simulink model "labFinal_5"  (R2018b)
settings: Solver=FixedStepDiscrete  StartTime=0.0  StopTime=10.0  FixedStep=1  RelTol=1e-3
libraries: hdlsllib x2
settings Model: Creator=mllax8  LastModifiedBy=mllax8

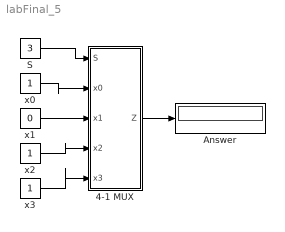
== system labFinal_5 ==
  4-1 MUX : Subsystem
  Answer : Display
  S : Constant  Value=3  OutDataTypeStr=uint8  SampleTime=1
  x0 : Constant  OutDataTypeStr=uint8  SampleTime=1
  x1 : Constant  Value=0  OutDataTypeStr=uint8  SampleTime=1
  x2 : Constant  OutDataTypeStr=uint8  SampleTime=1
  x3 : Constant  OutDataTypeStr=uint8  SampleTime=1
  wires:
  4-1 MUX/1(Z) -> Answer/1
  S/1 -> 4-1 MUX/1(S)
  x0/1 -> 4-1 MUX/2(x0)
  x1/1 -> 4-1 MUX/3(x1)
  x2/1 -> 4-1 MUX/4(x2)
  x3/1 -> 4-1 MUX/5(x3)

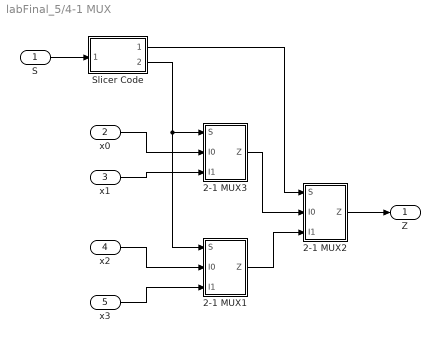
== system labFinal_5/4-1 MUX ==
  S : Inport  OutDataTypeStr=uint8
  x0 : Inport  Port=2  OutDataTypeStr=uint8
  x1 : Inport  Port=3  OutDataTypeStr=uint8
  x2 : Inport  Port=4  OutDataTypeStr=uint8
  x3 : Inport  Port=5  OutDataTypeStr=uint8
  2-1 MUX1 : Subsystem
  2-1 MUX2 : Subsystem
  2-1 MUX3 : Subsystem
  Slicer Code : Subsystem
  Z : Outport
  wires:
  Slicer Code/2("S 2^0 ") -> 2-1 MUX3/1(S), 2-1 MUX1/1(S)
  x0/1 -> 2-1 MUX3/2(I0)
  x1/1 -> 2-1 MUX3/3(I1)
  x2/1 -> 2-1 MUX1/2(I0)
  x3/1 -> 2-1 MUX1/3(I1)
  2-1 MUX3/1(Z) -> 2-1 MUX2/2(I0)
  2-1 MUX1/1(Z) -> 2-1 MUX2/3(I1)
  2-1 MUX2/1(Z) -> Z/1
  S/1 -> Slicer Code/1(uint8)
  Slicer Code/1(S 2^1) -> 2-1 MUX2/1(S)

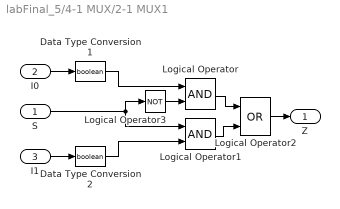
== system labFinal_5/4-1 MUX/2-1 MUX1 ==
  S : Inport
  I0 : Inport  Port=2
  I1 : Inport  Port=3
  Data Type Conversion1 : DataTypeConversion  OutDataTypeStr=boolean
  Data Type Conversion2 : DataTypeConversion  OutDataTypeStr=boolean
  Logical Operator : Logic  AllPortsSameDT=off  OutDataTypeStr=boolean
  Logical Operator1 : Logic  AllPortsSameDT=off  OutDataTypeStr=boolean
  Logical Operator2 : Logic  Operator=OR  AllPortsSameDT=off  OutDataTypeStr=boolean
  Logical Operator3 : Logic  Operator=NOT  AllPortsSameDT=off  OutDataTypeStr=boolean
  Z : Outport
  wires:
  Logical Operator2/1 -> Z/1
  I1/1 -> Data Type Conversion2/1
  Logical Operator1/1 -> Logical Operator2/2
  S/1 -> Logical Operator3/1, Logical Operator1/1
  I0/1 -> Data Type Conversion1/1
  Logical Operator/1 -> Logical Operator2/1
  Data Type Conversion1/1 -> Logical Operator/1
  Data Type Conversion2/1 -> Logical Operator1/2
  Logical Operator3/1 -> Logical Operator/2

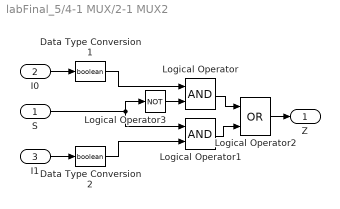
== system labFinal_5/4-1 MUX/2-1 MUX2 ==
  S : Inport
  I0 : Inport  Port=2
  I1 : Inport  Port=3
  Data Type Conversion1 : DataTypeConversion  OutDataTypeStr=boolean
  Data Type Conversion2 : DataTypeConversion  OutDataTypeStr=boolean
  Logical Operator : Logic  AllPortsSameDT=off  OutDataTypeStr=boolean
  Logical Operator1 : Logic  AllPortsSameDT=off  OutDataTypeStr=boolean
  Logical Operator2 : Logic  Operator=OR  AllPortsSameDT=off  OutDataTypeStr=boolean
  Logical Operator3 : Logic  Operator=NOT  AllPortsSameDT=off  OutDataTypeStr=boolean
  Z : Outport
  wires:
  Logical Operator2/1 -> Z/1
  I1/1 -> Data Type Conversion2/1
  Logical Operator1/1 -> Logical Operator2/2
  S/1 -> Logical Operator3/1, Logical Operator1/1
  I0/1 -> Data Type Conversion1/1
  Logical Operator/1 -> Logical Operator2/1
  Data Type Conversion1/1 -> Logical Operator/1
  Data Type Conversion2/1 -> Logical Operator1/2
  Logical Operator3/1 -> Logical Operator/2

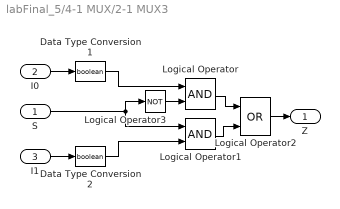
== system labFinal_5/4-1 MUX/2-1 MUX3 ==
  S : Inport
  I0 : Inport  Port=2
  I1 : Inport  Port=3
  Data Type Conversion1 : DataTypeConversion  OutDataTypeStr=boolean
  Data Type Conversion2 : DataTypeConversion  OutDataTypeStr=boolean
  Logical Operator : Logic  AllPortsSameDT=off  OutDataTypeStr=boolean
  Logical Operator1 : Logic  AllPortsSameDT=off  OutDataTypeStr=boolean
  Logical Operator2 : Logic  Operator=OR  AllPortsSameDT=off  OutDataTypeStr=boolean
  Logical Operator3 : Logic  Operator=NOT  AllPortsSameDT=off  OutDataTypeStr=boolean
  Z : Outport
  wires:
  Logical Operator2/1 -> Z/1
  I1/1 -> Data Type Conversion2/1
  Logical Operator1/1 -> Logical Operator2/2
  S/1 -> Logical Operator3/1, Logical Operator1/1
  I0/1 -> Data Type Conversion1/1
  Logical Operator/1 -> Logical Operator2/1
  Data Type Conversion1/1 -> Logical Operator/1
  Data Type Conversion2/1 -> Logical Operator1/2
  Logical Operator3/1 -> Logical Operator/2

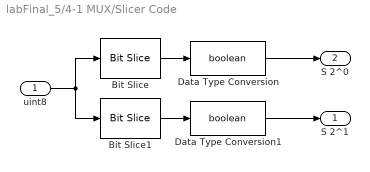
== system labFinal_5/4-1 MUX/Slicer Code ==
  uint8 : Inport  OutDataTypeStr=uint8  SampleTime=1
  Bit Slice : hdlsllib/Logic and Bit Operations/Bit Slice  lidx=0  ridx=0
  Bit Slice1 : hdlsllib/Logic and Bit Operations/Bit Slice  lidx=1  ridx=1
  Data Type Conversion : DataTypeConversion  OutDataTypeStr=boolean
  Data Type Conversion1 : DataTypeConversion  OutDataTypeStr=boolean
  S 2^1 : Outport
  "S 2^0 " : Outport  Port=2
  wires:
  Data Type Conversion1/1 -> S 2^1/1
  Data Type Conversion/1 -> "S 2^0 "/1
  Bit Slice1/1 -> Data Type Conversion1/1
  Bit Slice/1 -> Data Type Conversion/1
  uint8/1 -> Bit Slice/1, Bit Slice1/1
